simulink model "mymodel1"  (R2025b)
settings: Solver=VariableStepAuto  StartTime=0.0  StopTime=10.0  RelTol=1e-3
settings Model: Creator=VVK2GA  LastModifiedBy=VVK2GA

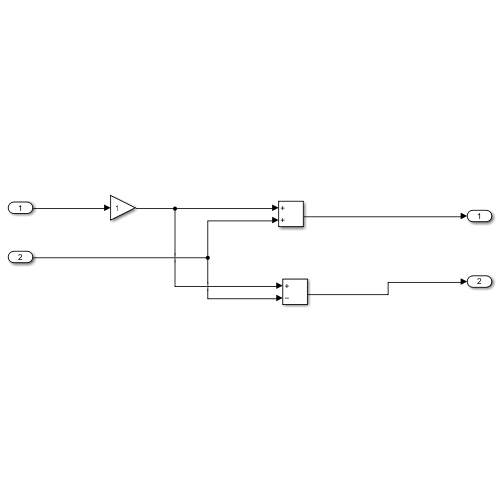
[thumbnail: Simulink's stored preview of the top-level diagram]
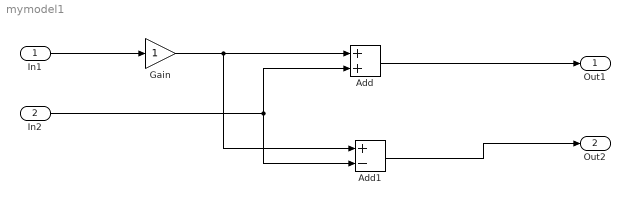
== system mymodel1 ==
  In1 : Inport
  In2 : Inport  Port=2
  Add : Sum
  Add1 : Sum  Inputs=+-
  Gain : Gain
  Out1 : Outport
  Out2 : Outport  Port=2
  wires:
  In1/1 -> Gain/1
  In2/1 -> Add1/2, Add/2
  Gain/1 -> Add1/1, Add/1
  Add/1 -> Out1/1
  Add1/1 -> Out2/1
